simulink model "main_RI_LIEKF_GNSSOutrage"  (R2023a)
settings: Solver=FixedStepAuto  StartTime=0.0  StopTime=220  FixedStep=0.01  RelTol=1e-3
InitFcn:
  | initNavigation0612_AOA;
values from neighbouring files (symbols this model uses):
  CF_enable = 0    [initNavigation.m]
  dt = 0.01    [initNavigation.m]
  dtDelay = -0.03    [initNavigation.m]
  g0 = 9.795    [initNavigation.m]
  gam0_rad = 0/57.3    (= 0)    [initNavigation.m]
  GNSSoutragetime = 90    [initNavigation.m]
  H_sensor_type = 0    [initNavigation.m]
  KF_enable = 1    [initNavigation.m]
  P0 = diag([1*ones(3,1);0.01*ones(3,1);0.1*ones(3,1);0.001*ones(3,1);0.00001*ones(3,1)])    [initNavigation.m]
  P0_RIEKF = diag([1*ones(3,1);0.01*ones(3,1);0.1*ones(3,1);0.001*ones(3,1);0.00001*ones(3,1);      0.01*ones(3,1);[0;2;2]/57.3;[0.1;0.1;0.1]])^2    [initNavigation.m]
  pd0 = 0    [initNavigation.m]
  pe0 = 0    [initNavigation.m]
  phi0_rad = 0/57.3    (= 0)    [initNavigation.m]
  pn0 = 0    [initNavigation.m]
  psi = -178    [initNavigation.m]
  psi0_rad = 0/57.3    (= 0)    [initNavigation.m]
  state_dim = 24    [initNavigation.m]
  Time = 0:0.01:(size(traindata.AttackAngle,1) - 1)*0.01    [NNLiftCoefficientFit.m]
  vd0 = 0    [initNavigation.m]
  ve0 = 0    [initNavigation.m]
  vn0 = 0    [initNavigation.m]
undefined symbols (not defined in the file or in its folder): DiscIntNeverNeededParam, Discrete, INS_CONST, INS_EXPORT, INS_PARAM, magnitude, p, param, pInitialization, sys
libraries: simulink_extras x94, simulink x82, dspstat3 x70, sharedtransform x60, ctrlSharedLib x36, sharedTrackingLibrary x22, matrix_library x15, FMT_Model_Lib x13, deeplib x8, dspsolvers x4, vrlib x4, aerolibconvert2 x1
(part 20 of 28)

== system main_RI_LIEKF_GNSSOutrage/State estimation/distribute CF/AHRS/Init_Q0/Horizontal_attitude ==
  note: gamma
  note: fai
  accl_mean_B_m/s_LPF : Inport  PortDimensions=3
  Magn_mean_B_guess_LPF : Inport  Port=2
  Enable : EnablePort
  Add : Sum  Inputs=+-
  Add1 : Sum
  Add2 : Sum
  Add3 : Sum
  Asin : Trigonometry  Operator=asin
  Atan2 : Trigonometry  Operator=atan2
  Data Type Conversion : DataTypeConversion  SaturateOnIntegerOverflow=off  RndMeth=Floor
  Deal with zero : Subsystem
  Degrees to Radians : simulink_extras/Transformations/Degrees to Radians
  Degrees to Radians1 : simulink_extras/Transformations/Degrees to Radians
  Demux : Demux  Outputs=3
  Divide : Product  Inputs=*/  OutDataTypeStr=single
  Gain1 : Gain  Gain=-1
  Gain2 : Gain  Gain=-1
  Magnetic declination : Constant  Value=param.fusion.magDeclDeg  OutDataTypeStr=single
  Magnetic declination1 : Constant  Value=param.control.MagnheadingCorrection  OutDataTypeStr=uint8
  Math Function : Math  Operator=magnitude^2  SignedPower=on
  Mux : Mux  Inputs=3
  Mux1 : Mux  Inputs=3
  Mux3 : Mux  Inputs=3
  Product : Product  Multiplication=Matrix(*)
  Quaternions to Direction Cosine Matrix : sharedtransform/Quaternions to  Direction Cosine Matrix  aMode=aMode
  Rotation Angles to Quaternions : sharedtransform/Rotation Angles to Quaternions  rotationOrder=ZYX  aMode=aMode
  Rotation Angles to Quaternions1 : sharedtransform/Rotation Angles to Quaternions  rotationOrder=ZYX  aMode=aMode
  Scope : Scope
  Scope1 : Scope
  Selector : Selector  InputPortWidth=3  IndexOptions=Index vector (dialog)  Indices=[2]  OutputSizes=1
  Selector1 : Selector  InputPortWidth=3  IndexOptions=Index vector (dialog)  Indices=[1]  OutputSizes=1
  Sqrt : Sqrt
  Sum of Elements : Sum  Inputs=+
  Switch : Switch  Threshold=0.5  SaturateOnIntegerOverflow=off  InputSameDT=off
  Terminator : Terminator
  Transpose : Math  Operator=transpose  SignedPower=on
  Trigonometric Function1 : Trigonometry  Operator=atan2
  psi_zero : Constant  Value=psi  OutDataTypeStr=single
  psi_zero1 : Constant  Value=psi0_rad  OutDataTypeStr=single
  psi_zero2 : Constant  Value=phi0_rad  OutDataTypeStr=single
  psi_zero3 : Constant  Value=gam0_rad  OutDataTypeStr=single
  quat_0 : Outport  PortDimensions=4
  wires:
  Data Type Conversion/1 -> Scope/1
  Rotation Angles to Quaternions1/1 -> Switch/1
  Switch/1 -> quat_0/1, Scope1/1
  Magnetic declination1/1 -> Switch/2, Data Type Conversion/1
  Degrees to Radians/1 -> Terminator/1
  Add1/1 -> Mux1/1
  Gain1/1 -> Mux/3, Trigonometric Function1/2
  Transpose/1 -> Product/1
  Mux3/1 -> Rotation Angles to Quaternions1/1
  Add/1 -> Mux3/1  "psi_calbymag"
  Magnetic declination/1 -> Degrees to Radians/1
  Atan2/1 -> Add/2
  Selector/1 -> Atan2/1  "magE"
  Selector1/1 -> Atan2/2  "magN"
  Product/1 -> Selector1/1, Selector/1  "magNED"
  Magn_mean_B_guess_LPF/1 -> Product/2
  Quaternions to Direction Cosine Matrix/1 -> Transpose/1
  Rotation Angles to Quaternions/1 -> Quaternions to Direction Cosine Matrix/1, Switch/3  "q0_no_yaw"
  Add3/1 -> Mux3/3, Mux1/3
  Add2/1 -> Mux1/2, Mux3/2
  psi_zero/1 -> Degrees to Radians1/1
  Mux1/1 -> Rotation Angles to Quaternions/1
  Math Function/1 -> Sum of Elements/1
  Mux/1 -> Math Function/1
  Divide/1 -> Asin/1
  Sum of Elements/1 -> Sqrt/1
  Demux/3 -> Gain1/1
  Demux/2 -> Trigonometric Function1/1, Mux/1
  Demux/1 -> Mux/2, Divide/1
  Trigonometric Function1/1 -> Gain2/1
  Deal with zero/1(Out1) -> Divide/2
  Sqrt/1 -> Deal with zero/1(In1)
  accl_mean_B_m/s_LPF/1 -> Demux/1
  psi_zero1/1 -> ?
  Degrees to Radians1/1 -> Add1/2
  psi_zero2/1 -> ?
  Asin/1 -> Add2/2
  psi_zero3/1 -> ?
  Gain2/1 -> Add3/2

== system main_RI_LIEKF_GNSSOutrage/State estimation/distribute CF/AHRS/Init_Q0/Subsystem ==
  data : Inport
  Buffer : Buffer  N=50  V=49  OutputFrames=off
  Buffer1 : Buffer  N=50  V=49  OutputFrames=off
  Buffer2 : Buffer  N=50  V=49  ic=-g0  OutputFrames=off
  Demux : Demux  Outputs=3
  Mean4 : dspstat3/Mean  run=off  reset_popup=None  directionMode=Entire input  dimension=3  roiEnable=off  roiType=Rectangles  roiPortion=Entire ROI  roiOutput=Individual statistics for each ROI  roiFlag=off  roundingMode=Floor  overflowMode=off  outputDataTypeStr=Inherit: Same as accumulator  outputMin=[]  outputMax=[]  outputLastDataTypeStr=Inherit: Same as accumulator
  Mean5 : dspstat3/Mean  run=off  reset_popup=None  directionMode=Entire input  dimension=3  roiEnable=off  roiType=Rectangles  roiPortion=Entire ROI  roiOutput=Individual statistics for each ROI  roiFlag=off  roundingMode=Floor  overflowMode=off  outputDataTypeStr=Inherit: Same as accumulator  outputMin=[]  outputMax=[]  outputLastDataTypeStr=Inherit: Same as accumulator
  Mean6 : dspstat3/Mean  run=off  reset_popup=None  directionMode=Entire input  dimension=3  roiEnable=off  roiType=Rectangles  roiPortion=Entire ROI  roiOutput=Individual statistics for each ROI  roiFlag=off  roundingMode=Floor  overflowMode=off  outputDataTypeStr=Inherit: Same as accumulator  outputMin=[]  outputMax=[]  outputLastDataTypeStr=Inherit: Same as accumulator
  Scope : Scope  NumInputPorts=2
  Vector Concatenate : Concatenate  NumInputs=3
  mean_data : Outport
  wires:
  data/1 -> Demux/1, Scope/1
  Vector Concatenate/1 -> mean_data/1, Scope/2
  Mean4/1 -> Vector Concatenate/1
  Demux/3 -> Buffer2/1
  Buffer1/1 -> Mean5/1  "fby_buff"
  Demux/1 -> Buffer/1
  Buffer2/1 -> Mean6/1  "fbz_buff"
  Mean5/1 -> Vector Concatenate/2
  Buffer/1 -> Mean4/1  "fbx_buff"
  Demux/2 -> Buffer1/1
  Mean6/1 -> Vector Concatenate/3

== system main_RI_LIEKF_GNSSOutrage/State estimation/distribute CF/AHRS/Init_Q0/Subsystem1 ==
  data : Inport
  Buffer : Buffer  N=50  V=49  OutputFrames=off
  Buffer1 : Buffer  N=50  V=49  OutputFrames=off
  Buffer2 : Buffer  N=50  V=49  OutputFrames=off
  Demux : Demux  Outputs=3
  Mean4 : dspstat3/Mean  run=off  reset_popup=None  directionMode=Entire input  dimension=3  roiEnable=off  roiType=Rectangles  roiPortion=Entire ROI  roiOutput=Individual statistics for each ROI  roiFlag=off  roundingMode=Floor  overflowMode=off  outputDataTypeStr=Inherit: Same as accumulator  outputMin=[]  outputMax=[]  outputLastDataTypeStr=Inherit: Same as accumulator
  Mean5 : dspstat3/Mean  run=off  reset_popup=None  directionMode=Entire input  dimension=3  roiEnable=off  roiType=Rectangles  roiPortion=Entire ROI  roiOutput=Individual statistics for each ROI  roiFlag=off  roundingMode=Floor  overflowMode=off  outputDataTypeStr=Inherit: Same as accumulator  outputMin=[]  outputMax=[]  outputLastDataTypeStr=Inherit: Same as accumulator
  Mean6 : dspstat3/Mean  run=off  reset_popup=None  directionMode=Entire input  dimension=3  roiEnable=off  roiType=Rectangles  roiPortion=Entire ROI  roiOutput=Individual statistics for each ROI  roiFlag=off  roundingMode=Floor  overflowMode=off  outputDataTypeStr=Inherit: Same as accumulator  outputMin=[]  outputMax=[]  outputLastDataTypeStr=Inherit: Same as accumulator
  Vector Concatenate : Concatenate  NumInputs=3
  mean_data : Outport
  wires:
  Mean6/1 -> Vector Concatenate/3
  Demux/2 -> Buffer1/1
  Buffer/1 -> Mean4/1  "fbx_buff"
  Mean5/1 -> Vector Concatenate/2
  Buffer2/1 -> Mean6/1  "fbz_buff"
  Demux/1 -> Buffer/1
  Buffer1/1 -> Mean5/1  "fby_buff"
  Demux/3 -> Buffer2/1
  Mean4/1 -> Vector Concatenate/1
  Vector Concatenate/1 -> mean_data/1
  data/1 -> Demux/1

== system main_RI_LIEKF_GNSSOutrage/State estimation/distribute CF/AHRS/att_update/uniformization ==
  Q i : Inport  PortDimensions=4
  Constant : Constant  Value=1e-20
  Dot Product1 : DotProduct  OutDataTypeStr=Inherit: Inherit via internal rule
  Math Function : Math  Operator=sqrt  SignedPower=on
  Product : Product  Inputs=*/  SaturateOnIntegerOverflow=on  OutDataTypeStr=Inherit: Same as first input
  Sum : Sum  Inputs=|++  SaturateOnIntegerOverflow=on
  Q o : Outport
  wires:
  Sum/1 -> Product/2
  Constant/1 -> Sum/2
  Product/1 -> Q o/1
  Math Function/1 -> Sum/1
  Dot Product1/1 -> Math Function/1
  Q i/1 -> Product/1, Dot Product1/1, Dot Product1/2

== system main_RI_LIEKF_GNSSOutrage/State estimation/distribute CF/Translation_estimate/Rxy_Horizontal_estimation/Integrator_R_Horizontal ==
  Vn : Inport
  dR : Inport  Port=2
  Sensor_data2 : Inport  Port=3
  Bus Selector : BusSelector  OutputSignals=QGC_sensor_reinit,GPS_Data.pos_N_gps,GPS_Data.pos_E_gps
  Delay : Delay  DelayLength=1  InitialConditionSource=Input port  ExternalReset=Rising
      settings: InputPortMap=u0,r5,p4
  Gain : Gain  Gain=0.8
  Gain2 : Gain  Gain=dt  SaturateOnIntegerOverflow=on  OutDataTypeStr=Inherit: Same as input  ParamDataTypeStr=Inherit: Same as input
  Mux : Mux  Inputs=2
  Sum : Sum  Inputs=|++-
  R_n&e : Outport
  wires:
  Gain/1 -> Sum/3
  dR/1 -> Gain/1
  Vn/1 -> Gain2/1
  Gain2/1 -> Sum/1
  Sum/1 -> R_n&e/1, Delay/1
  Sensor_data2/1 -> Bus Selector/1
  Bus Selector/1 -> Delay/2  "<QGC_sensor_reinit>"
  Bus Selector/2 -> Mux/1  "<pos_N_gps>"
  Bus Selector/3 -> Mux/2  "<pos_E_gps>"
  Mux/1 -> Delay/3
  Delay/1 -> Sum/2

== system main_RI_LIEKF_GNSSOutrage/State estimation/distribute CF/Translation_estimate/Rxy_Horizontal_estimation/Rxy_kalman filter2 ==
  X : Inport
  Z : Inport  Port=2
  Enable : Inport  Port=3
  Constant : Constant  Value=F  OutDataTypeStr=single
  Constant1 : Constant  Value=Q  OutDataTypeStr=single
  Constant2 : Constant  Value=R  OutDataTypeStr=single
  Constant3 : Constant  Value=P0  OutDataTypeStr=single
  Constant4 : Constant  Value=H  OutDataTypeStr=single
  Vxy kalman filter : Subsystem  TreatAsAtomicUnit=on
  XOut : Outport
  wires:
  Enable/1 -> Vxy kalman filter/9(Enable)
  Vxy kalman filter/1(XOut) -> XOut/1
  Constant1/1 -> Vxy kalman filter/5(Q)
  Constant4/1 -> Vxy kalman filter/4(H)
  Constant2/1 -> Vxy kalman filter/6(R)
  Constant3/1 -> Vxy kalman filter/8(P0)
  Z/1 -> Vxy kalman filter/1(Z)
  Constant/1 -> Vxy kalman filter/3(G), Vxy kalman filter/2(F)
  X/1 -> Vxy kalman filter/7(X)

== system main_RI_LIEKF_GNSSOutrage/State estimation/distribute CF/Translation_estimate/V_Horizontal_estimation/Integrator_V_Horizontal ==
  An : Inport
  dv : Inport  Port=2
  Sensor_data2 : Inport  Port=3
  Bus Selector : BusSelector  OutputSignals=QGC_sensor_reinit,GPS_Data.vn_gps,GPS_Data.ve_gps
  Delay : Delay  DelayLength=1  InitialConditionSource=Input port  ExternalReset=Rising
      settings: InputPortMap=u0,r5,p4
  Gain : Gain
  Gain2 : Gain  Gain=dt  SaturateOnIntegerOverflow=on  OutDataTypeStr=Inherit: Same as input  ParamDataTypeStr=Inherit: Same as input
  Mux : Mux  Inputs=2
  Scope : Scope
  Sum : Sum  Inputs=|++-
  V_n&e : Outport
  wires:
  Gain/1 -> Sum/3, Scope/1
  dv/1 -> Gain/1
  Delay/1 -> Sum/2
  Mux/1 -> Delay/3
  Bus Selector/3 -> Mux/2  "<ve_gps>"
  Bus Selector/2 -> Mux/1  "<vn_gps>"
  Bus Selector/1 -> Delay/2  "<QGC_sensor_reinit>"
  Sensor_data2/1 -> Bus Selector/1
  Sum/1 -> Delay/1, V_n&e/1
  Gain2/1 -> Sum/1
  An/1 -> Gain2/1

== system main_RI_LIEKF_GNSSOutrage/State estimation/distribute CF/Translation_estimate/V_Horizontal_estimation/Rxy_kalman filter1 ==
  X : Inport
  Z : Inport  Port=2
  Enable : Inport  Port=3
  Constant : Constant  Value=F  OutDataTypeStr=single
  Constant1 : Constant  Value=Q  OutDataTypeStr=single
  Constant2 : Constant  Value=R  OutDataTypeStr=single
  Constant3 : Constant  Value=P0  OutDataTypeStr=single
  Constant4 : Constant  Value=H  OutDataTypeStr=single
  Vxy kalman filter : Subsystem  TreatAsAtomicUnit=on
  XOut : Outport
  wires:
  X/1 -> Vxy kalman filter/7(X)
  Constant/1 -> Vxy kalman filter/2(F), Vxy kalman filter/3(G)
  Z/1 -> Vxy kalman filter/1(Z)
  Constant3/1 -> Vxy kalman filter/8(P0)
  Constant2/1 -> Vxy kalman filter/6(R)
  Constant4/1 -> Vxy kalman filter/4(H)
  Constant1/1 -> Vxy kalman filter/5(Q)
  Vxy kalman filter/1(XOut) -> XOut/1
  Enable/1 -> Vxy kalman filter/9(Enable)

== system main_RI_LIEKF_GNSSOutrage/State estimation/distribute CF/distribute CF/AHRS1/Bus_Constructor ==
  RF_Data : Inport
  att_quat : Inport  Port=2
  DCM_OB : Inport  Port=3
  bias_g : Inport  Port=4
  Sensor_Data : Inport  Port=5
  Bus Creator : BusCreator  Inputs=12
  Bus Selector : BusSelector  OutputSignals=IMU_Data.gyr_B_radPs,IMU_Data.acc_B_mPs2
  Bus Selector1 : BusSelector  OutputSignals=att_reset
  Bus Selector2 : BusSelector  OutputSignals=standstill
  Euler_Angle : Subsystem
  Math Function : Math  Operator=transpose  SignedPower=on
  Psi To DCM : FMT_Model_Lib/Transformation/Psi To DCM
  Signal Conversion{,1..4} (5 alike) : SignalConversion  OverrideOpt=off
  Rotation_Data : Outport
  wires:
  Bus Selector1/1 -> Signal Conversion4/1  "<att_reset>"
  Signal Conversion/1 -> Bus Creator/11  "acc_B_mPs2"
  Euler_Angle/1(phi_rad) -> Bus Creator/2  "phi_rad"
  Euler_Angle/2(theta_rad) -> Bus Creator/3  "theta_rad"
  Euler_Angle/3(psi_rad) -> Psi To DCM/1, Bus Creator/4  "psi_rad"
  Sensor_Data/1 -> Bus Selector/1
  Bus Selector2/1 -> Signal Conversion1/1  "<standstill>"
  Bus Creator/1 -> Rotation_Data/1
  bias_g/1 -> Signal Conversion3/1
  Math Function/1 -> Bus Creator/7  "M_BO"
  DCM_OB/1 -> Math Function/1, Bus Creator/8  "M_OB"
  att_quat/1 -> Euler_Angle/1(att_quat), Bus Creator/6  "att_quat"
  Psi To DCM/1 -> Bus Creator/5  "M_CO"
  Signal Conversion1/1 -> Bus Creator/12  "standstill"
  Bus Selector/2 -> Signal Conversion/1  "<acc_B_mPs2>"
  Signal Conversion2/1 -> Bus Creator/10  "gyr_B_radPs"
  Signal Conversion3/1 -> Bus Creator/9  "bias_g"
  RF_Data/1 -> Bus Selector2/1, Bus Selector1/1  "att_reset"
  Bus Selector/1 -> Signal Conversion2/1  "<gyr_B_radPs>"
  Signal Conversion4/1 -> Bus Creator/1  "att_reset"

== system main_RI_LIEKF_GNSSOutrage/State estimation/distribute CF/distribute CF/AHRS1/Correct ==
  Rotation_Data : Inport
  Sensor_Data : Inport  Port=2
  RF_Data : Inport  Port=3
  Attitude_Correction : Subsystem
  Bus Selector : BusSelector  OutputSignals=standstill
  Bus Selector1 : BusSelector  OutputSignals=IMU_Data
  Gyro_Bias_Correction : Subsystem
  att_B_correction : Outport
  bias_g_B_correction : Outport  Port=2
  wires:
  Gyro_Bias_Correction/1(bias_g_B_correction) -> bias_g_B_correction/1
  Bus Selector1/1 -> Gyro_Bias_Correction/2(IMU_Data)  "<IMU_Data>"
  RF_Data/1 -> Bus Selector/1
  Attitude_Correction/1(att_B_correction) -> att_B_correction/1, Gyro_Bias_Correction/1(att_B_correction)
  Sensor_Data/1 -> Attitude_Correction/1(Sensor_Data), Bus Selector1/1
  Rotation_Data/1 -> Attitude_Correction/2(Rotation_Data)
  Bus Selector/1 -> Attitude_Correction/3(standstill)  "<standstill>"

== system main_RI_LIEKF_GNSSOutrage/State estimation/distribute CF/distribute CF/AHRS1/Update ==
  att_B_correction : Inport
  bias_g_correction : Inport  Port=2
  RF_Data : Inport  Port=3
  Sensor_Data : Inport  Port=4
  Attitude_Update : Subsystem
  Bus Selector : BusSelector  OutputSignals=IMU_Data.gyr_B_radPs
  Bus Selector1 : BusSelector  OutputSignals=att_reset,quat_0
  Gyro_Bias_Update : Subsystem
  Sum2 : Sum  Inputs=|++
  att_quat : Outport
  DCM_OB : Outport  Port=2
  bias_g : Outport  Port=3
  wires:
  Sensor_Data/1 -> Bus Selector/1
  Gyro_Bias_Update/1(gyr_B_correction) -> Sum2/2
  att_B_correction/1 -> Sum2/1
  Sum2/1 -> Attitude_Update/3(att_B_correction)
  Bus Selector/1 -> Gyro_Bias_Update/2(gyr_B_radPs)  "<gyr_B_radPs>"
  bias_g_correction/1 -> Gyro_Bias_Update/1(bias_g_correction)
  Attitude_Update/1(att_quat) -> att_quat/1
  Attitude_Update/2(DCM_OB) -> DCM_OB/1
  Gyro_Bias_Update/2(bias_g) -> bias_g/1
  RF_Data/1 -> Bus Selector1/1  "att_reset"
  Bus Selector1/1 -> Attitude_Update/1(att_reset)  "<att_reset>"
  Bus Selector1/2 -> Attitude_Update/2(quat_0)  "<quat_0>"

== system main_RI_LIEKF_GNSSOutrage/State estimation/distribute CF/distribute CF/Bus_Constructor/Euler_Angle ==
  att_quat : Inport
  Demux : Demux  Outputs=3
  Quaternions to Rotation Angles : sharedtransform/Quaternions to Rotation Angles  rotationOrder=ZYX  aMode=aMode
  phi_rad : Outport
  theta_rad : Outport  Port=2
  psi_rad : Outport  Port=3
  wires:
  Demux/1 -> phi_rad/1
  Demux/2 -> theta_rad/1
  Demux/3 -> psi_rad/1
  att_quat/1 -> Quaternions to Rotation Angles/1
  Quaternions to Rotation Angles/1 -> Demux/1

== system main_RI_LIEKF_GNSSOutrage/State estimation/distribute CF/distribute CF/Bus_Constructor/Subsystem1 ==
  psi : Inport
  Gain : Gain  Gain=-1
  Subsystem : Subsystem
  DCMz : Outport
  wires:
  psi/1 -> Gain/1
  Gain/1 -> Subsystem/1(psi)
  Subsystem/1(DCMz) -> DCMz/1

== system main_RI_LIEKF_GNSSOutrage/State estimation/distribute CF/distribute CF/Correct/Attitude_Correction ==
  note: N系到B系
  Sensor_Data : Inport
  Rotation_Data : Inport  Port=2
  Attitude_Correct : Subsystem
  Bus Selector2 : BusSelector  OutputSignals=M_BO
  Mag_Correct : Subsystem
  Multiply : Product  Multiplication=Matrix(*)
  Scope : Scope
  Sum : Sum  Inputs=|++
  att_B_correction : Outport
  wires:
  Multiply/1 -> att_B_correction/1
  Rotation_Data/1 -> Bus Selector2/1, Attitude_Correct/2(Rotation_Data), Mag_Correct/1(Rotation_Data)
  Sensor_Data/1 -> Mag_Correct/2(Sensor_Data), Attitude_Correct/1(Sensor_Data)
  Bus Selector2/1 -> Multiply/1  "<M_BO>"
  Sum/1 -> Multiply/2
  Attitude_Correct/1(att_corr_O) -> Sum/1
  Mag_Correct/1(mag_corr_O) -> Scope/1  "mag_corr_O"

== system main_RI_LIEKF_GNSSOutrage/State estimation/distribute CF/distribute CF/Correct/Subsystem2 ==
  note: 零速判断
  note: 误差角r
  note: 误差角速度r‘
  Sensor_Data : Inport
  att_B_correction : Inport  Port=2
  Abs : Abs  SaturateOnIntegerOverflow=off
  Bus Selector1 : BusSelector  OutputSignals=IMU_Data.accl_B_m/s2_LPF
  Compare To Constant : simulink/Logic and Bit Operations/Compare To Constant  relop=<=  const=1  OutDataTypeStr=boolean
  Constant : Constant  Value=g0  OutDataTypeStr=single
  Data Type Conversion : DataTypeConversion  OutDataTypeStr=single  SaturateOnIntegerOverflow=off  RndMeth=Floor
  Gain1 : Gain  Gain=gbias_correct_gain
  MX Product1 : Product  RndMeth=Simplest
  Saturation2 : Saturate  UpperLimit=0.1/180*pi  LowerLimit=-0.1/180*pi
  Scope : Scope
  Scope1 : Scope  NumInputPorts=2
  Subtract : Sum  Inputs=+-
  norm : Subsystem
  低通滤波 : Subsystem  mask{fc=5, zeta=0.707}
      mask prompts: fc "Cut-off frequence"; zeta "Damping factor"
      mask DialogControl ParameterGroupVar Prompt: 参数
  bias_g_B_correction : Outport
  wires:
  Sensor_Data/1 -> Bus Selector1/1
  Saturation2/1 -> bias_g_B_correction/1  "bias_g_correction"
  Constant/1 -> Subtract/2
  Compare To Constant/1 -> Data Type Conversion/1
  att_B_correction/1 -> MX Product1/1
  Data Type Conversion/1 -> Scope/1, MX Product1/2
  MX Product1/1 -> Scope1/1, 低通滤波/1(u)
  Subtract/1 -> Abs/1
  norm/1(Out1) -> Subtract/1
  Bus Selector1/1 -> norm/1(In1)  "<accl_B_m/s2_LPF>"
  Abs/1 -> Compare To Constant/1
  Gain1/1 -> Saturation2/1
  低通滤波/1(y) -> Scope1/2, Gain1/1

== system main_RI_LIEKF_GNSSOutrage/State estimation/distribute CF/distribute CF/Translation_estimate/Rxy_Horizontal_estimation ==
  Vn : Inport
  Enable : Inport  Port=2
  Sensor_data2 : Inport  Port=3
  Cbn : Inport  Port=4
  Add1 : Sum  Inputs=+-
  Bus Selector1 : BusSelector  OutputSignals=GPS_Data.pos_N_gps,GPS_Data.pos_E_gps
  Data Store Memory : DataStoreMemory  DataStoreName=GPS_enable_CF  WriteAfterWriteMsg=warning  ShowAdditionalParam=off
  Data Store Read : DataStoreRead  DataStoreName=GPS_enable_CF  IndexOptions=Index vector (dialog)  Indices=1  OutputSizes=1
  Data Store Write : DataStoreWrite  DataStoreName=GPS_enable_CF  IndexOptions=Index vector (dialog)  Indices=1  OutputSizes=1
  Delay1 : Delay  DelayLength=1
  Integrator_R_Horizontal : Subsystem
  Mux1 : Mux  Inputs=2
  Rxy_kalman filter2 : Subsystem  mask{F=diag([-0.1,-0.1,-0.01,-0.01]), H=[1,0,-1,0;0,1,0,-1], Q=diag([1,1,0.1,0.1]), R=diag([0.05,0.05]), P0=diag([0.8,0.8,0.2,0.2])}
      mask prompts: F "状态转移矩阵：F"; H "观测转移矩阵：H"; Q "预测噪声协方差矩阵：Q"; R "量测噪声协方差矩阵：R"; P0 "初始协方差矩阵：P0"
      mask DialogControl DescTextVar Prompt: Kalman Filter
  Scope : Scope
  Scope1 : Scope  NumInputPorts=2
  Scope5 : Scope
  Selector1 : Selector  InputPortWidth=4  IndexOptions=Index vector (dialog)  Indices=[1 2]  OutputSizes=1
  Subsystem : Subsystem
  R_n&e : Outport
  wires:
  Vn/1 -> Integrator_R_Horizontal/1(Vn)
  Add1/1 -> Rxy_kalman filter2/2(Z)
  Rxy_kalman filter2/1(XOut) -> Scope/1, Delay1/1
  Bus Selector1/1 -> Mux1/1  "<pos_N_gps>"
  Integrator_R_Horizontal/1(R_n&e) -> R_n&e/1
  Bus Selector1/2 -> Mux1/2  "<pos_E_gps>"
  Sensor_data2/1 -> Bus Selector1/1, Integrator_R_Horizontal/3(Sensor_data2)
  Delay1/1 -> Rxy_kalman filter2/1(X), Selector1/1
  Mux1/1 -> Scope1/2, Add1/2
  Selector1/1 -> Integrator_R_Horizontal/2(dR)
  Cbn/1 -> Integrator_R_Horizontal/4(Cbn)
  Integrator_R_Horizontal/2(R_n&eL) -> Scope1/1, Add1/1
  Subsystem/1(flag) -> Scope5/1, Data Store Write/1
  Data Store Read/1 -> Rxy_kalman filter2/3(Enable)

== system main_RI_LIEKF_GNSSOutrage/State estimation/distribute CF/distribute CF/Translation_estimate/V_Horizontal_estimation ==
  note: 0530改：
      | 加入GPStype限制
  An : Inport
  Sensor_data2 : Inport  Port=2
  Add : Sum  Inputs=+-
  Bus Selector2 : BusSelector  OutputSignals=GPS_Data.vn_gps,GPS_Data.ve_gps,GPS_Data.fixtype_gps
  Compare To Constant : simulink/Logic and Bit Operations/Compare To Constant  relop=>=  const=1  OutDataTypeStr=boolean
  Delay : Delay  DelayLength=1
  Detect Change : simulink/Logic and Bit Operations/Detect Change  vinit=0  OutDataTypeStr=boolean
  Integrator_V_Horizontal : Subsystem
  Logical Operator : Logic  AllPortsSameDT=off  OutDataTypeStr=boolean
  Mux : Mux  Inputs=2
  Rxy_kalman filter1 : Subsystem  mask{F=diag([-0.1,-0.1,-0.01,-0.01]), H=[1,0,-1,0;0,1,0,-1], Q=diag([1,1,0.1,0.1]), R=diag([0.1,0.1]), P0=diag([0.8,0.8,0.5,0.5])}
      mask prompts: F "状态转移矩阵：F"; H "观测转移矩阵：H"; Q "预测噪声协方差矩阵：Q"; R "量测噪声协方差矩阵：R"; P0 "初始协方差矩阵：P0"
      mask DialogControl DescTextVar Prompt: Kalman Filter
  Scope : Scope  NumInputPorts=2
  Scope1 : Scope
  Selector : Selector  InputPortWidth=4  IndexOptions=Index vector (dialog)  Indices=[1 2]  OutputSizes=1
  vxy_estimout : Outport
  V_n&e : Outport  Port=2
  GPS_v_enable : Outport  Port=3
  wires:
  Logical Operator/1 -> Rxy_kalman filter1/3(Enable), GPS_v_enable/1, Scope1/1
  Compare To Constant/1 -> Logical Operator/2
  Detect Change/1 -> Logical Operator/1
  Bus Selector2/3 -> Compare To Constant/1  "<fixtype_gps>"
  Sensor_data2/1 -> Integrator_V_Horizontal/3(Sensor_data2), Bus Selector2/1
  An/1 -> Integrator_V_Horizontal/1(An)
  Add/1 -> Rxy_kalman filter1/2(Z)
  Integrator_V_Horizontal/1(V_n&e) -> Add/1, Scope/1, vxy_estimout/1, V_n&e/1
  Rxy_kalman filter1/1(XOut) -> Delay/1
  Bus Selector2/2 -> Mux/2  "<ve_gps>"
  Mux/1 -> Add/2, Scope/2
  Bus Selector2/1 -> Detect Change/1, Mux/1  "<vn_gps>"
  Selector/1 -> Integrator_V_Horizontal/2(dv)
  Delay/1 -> Rxy_kalman filter1/1(X), Selector/1

== system main_RI_LIEKF_GNSSOutrage/State estimation/distribute CF/distribute CF/Translation_estimate/translate to N ==
  RotationData : Inport
  Sensor_data : Inport  Port=2
  Bus Selector2 : BusSelector  OutputSignals=IMU_Data.accl_B_m/s2_LPF
  Bus Selector3 : BusSelector  OutputSignals=M_OB
  Product : Product  Multiplication=Matrix(*)
  Selector : Selector  InputPortWidth=3  IndexOptions=Index vector (dialog)  Indices=[1 2]  OutputSizes=1
  Selector1 : Selector  InputPortWidth=3  IndexOptions=Index vector (dialog)  Indices=[3]  OutputSizes=1
  accel_Horizontal_predict : Outport
  accel_Vertical_predict : Outport  Port=2
  wires:
  Selector1/1 -> accel_Vertical_predict/1
  Selector/1 -> accel_Horizontal_predict/1
  Product/1 -> Selector/1, Selector1/1
  Sensor_data/1 -> Bus Selector2/1
  Bus Selector3/1 -> Product/1  "<M_OB>"
  Bus Selector2/1 -> Product/2  "<accl_B_m/s2_LPF>"
  RotationData/1 -> Bus Selector3/1

== system main_RI_LIEKF_GNSSOutrage/State estimation/distribute CF/distribute CF/Update/Attitude_Update ==
  att_reset : Inport
  quat_0 : Inport  Port=2
  att_B_correction : Inport  Port=3
  Delay : Delay  DelayLength=1  InitialConditionSource=Input port  ExternalReset=Rising
      settings: InputPortMap=u0,r5,p4
  Gain : Gain  Gain=dt
  QuatMult1 : MATLAB Function  TreatAsAtomicUnit=on
  Quaternions to Direction Cosine Matrix1 : sharedtransform/Quaternions to  Direction Cosine Matrix  aMode=aMode
  Transpose1 : Math  Operator=transpose  SignedPower=on
  rv2q : MATLAB Function  TreatAsAtomicUnit=on
  uniformization1 : Subsystem
  att_quat : Outport
  DCM_OB : Outport  Port=2
  wires:
  Transpose1/1 -> DCM_OB/1  "DCM_b_n"
  rv2q/1(quaternion) -> QuatMult1/2(quatB)
  uniformization1/1(Q o) -> att_quat/1, Delay/1, Quaternions to Direction Cosine Matrix1/1  "q_update"
  Gain/1 -> rv2q/1(rotVec)  "correctedDelAng"
  Delay/1 -> QuatMult1/1(quatA)
  att_B_correction/1 -> Gain/1
  Quaternions to Direction Cosine Matrix1/1 -> Transpose1/1
  QuatMult1/1(quatOut) -> uniformization1/1(Q i)  "q_update"
  att_reset/1 -> Delay/2
  quat_0/1 -> Delay/3

== system main_RI_LIEKF_GNSSOutrage/State estimation/distribute CF/distribute CF/Update/Gyro_Bias_Update ==
  bias_g_correction : Inport
  gyr_B_radPs : Inport  Port=2
  Discrete-Time Integrator2 : DiscreteIntegrator  gainval=1  SampleTime=-1  LimitOutput=on  UpperSaturationLimit=45/180*pi  LowerSaturationLimit=-45/180*pi  ICPrevOutput=DiscIntNeverNeededParam  ICPrevScaledInput=DiscIntNeverNeededParam
  Sum1 : Sum  Inputs=++|
  gyr_B_correction : Outport
  bias_g : Outport  Port=2
  wires:
  Discrete-Time Integrator2/1 -> Sum1/1, bias_g/1
  gyr_B_radPs/1 -> Sum1/2
  Sum1/1 -> gyr_B_correction/1
  bias_g_correction/1 -> Discrete-Time Integrator2/1

== system main_RI_LIEKF_GNSSOutrage/State estimation/distribute CF/distribute CF/初始化/Attitude_Reset ==
  Sensor_Data : Inport
  Bus Selector : BusSelector  OutputSignals=IMU_Data.accl_B_m/s2_LPF
  Bus Selector1 : BusSelector  OutputSignals=GPS_Data.fixtype_gps
  Detect Rise Positive : simulink/Logic and Bit Operations/Detect Rise Positive  vinit=0  OutDataTypeStr=boolean
  Interval Test : simulink/Logic and Bit Operations/Interval Test  IntervalClosedRight=on  uplimit=g0+0.5  IntervalClosedLeft=on  lowlimit=g0-0.5  OutDataTypeStr=boolean
  Logical Operator : Logic  AllPortsSameDT=off  OutDataTypeStr=boolean
  Logical Operator2 : Logic  Operator=OR  AllPortsSameDT=off  OutDataTypeStr=boolean
  Reset Heading : Subsystem
  norm : Subsystem
  sample_valid : Subsystem
  att_reset : Outport
  wires:
  sample_valid/1(sample_valid) -> Logical Operator/1, Detect Rise Positive/1
  norm/1(Out1) -> Interval Test/1
  Interval Test/1 -> sample_valid/1(valid)
  Sensor_Data/1 -> Bus Selector1/1, Bus Selector/1
  Bus Selector/1 -> norm/1(In1)  "<accl_B_m/s2_LPF>"
  Detect Rise Positive/1 -> Logical Operator2/1
  Logical Operator/1 -> Logical Operator2/2
  Logical Operator2/1 -> att_reset/1
  Bus Selector1/1 -> Reset Heading/1(GPS_valid)  "<fixtype_gps>"
  Reset Heading/1(reset) -> Logical Operator/2

== system main_RI_LIEKF_GNSSOutrage/State estimation/distribute CF/distribute CF/初始化/Subsystem ==
  sensor_data : Inport
  Enable : EnablePort
  Bus Selector1 : BusSelector  OutputSignals=IMU_Data.accl_B_m/s2_LPF,MAGN_Data.mag_norm_B
  Cross Product2 : vrlib/Utilities/Cross Product
  Cross Product3 : vrlib/Utilities/Cross Product
  Direction Cosine Matrix to Quaternions : sharedtransform/Direction Cosine Matrix  to Quaternions  aMode=aMode  action=None  tolerance=eps(2)
  Gain : Gain  Gain=-1
  Normalized1 : Subsystem
  Normalized2 : Subsystem
  Normalized3 : Subsystem
  Vector Concatenate : Concatenate  NumInputs=3  Mode=Multidimensional array  ConcatenateDimension=2
  quat_0 : Outport
  wires:
  Gain/1 -> Cross Product2/1, Cross Product3/2, Normalized3/1(fb)
  Normalized2/1(fb/g) -> Vector Concatenate/2
  Normalized3/1(fb/g) -> Vector Concatenate/3
  Cross Product2/1 -> Cross Product3/1, Normalized2/1(fb)
  Vector Concatenate/1 -> Direction Cosine Matrix to Quaternions/1
  Normalized1/1(fb/g) -> Vector Concatenate/1
  Direction Cosine Matrix to Quaternions/1 -> quat_0/1
  Bus Selector1/2 -> Cross Product2/2  "<mag_norm_B>"
  Bus Selector1/1 -> Gain/1  "<accl_B_m/s2_LPF>"
  sensor_data/1 -> Bus Selector1/1
  Cross Product3/1 -> Normalized1/1(fb)

== system main_RI_LIEKF_GNSSOutrage/Sensor_Data_Process/Magn_Data_Process1/Mag_Data_Process/Mag_Quality_Estimate/Mag_Quality/Inclination_Quality_Estimate ==
  nominal_inc_deg : Inport
  mag_normalized_O : Inport  Port=2
  Abs1 : Abs  SaturateOnIntegerOverflow=off
  Constant2 : Constant  OutDataTypeStr=Inherit: Inherit via back propagation
  Gain1 : Gain  Gain=pi/180
  Norm(x) : Subsystem
  Saturation : Saturate  UpperLimit=1  LowerLimit=0
  Selector : Selector  InputPortWidth=3  IndexOptions=Index vector (dialog)  Indices=[1 2]  OutputSizes=1
  Selector1 : Selector  InputPortWidth=3  IndexOptions=Index vector (dialog)  Indices=3  OutputSizes=1
  Subtract : Sum  Inputs=+-
  Sum3 : Sum  Inputs=+-|
  Trigonometric Function : Trigonometry  Operator=atan2
  gain : Gain  Gain=2
  inclination_quality : Outport  VectorParamsAs1DForOutWhenUnconnected=off
  wires:
  mag_normalized_O/1 -> Selector1/1, Selector/1
  Trigonometric Function/1 -> Subtract/2
  Norm(x)/1(Out1) -> Trigonometric Function/2
  Abs1/1 -> gain/1
  gain/1 -> Sum3/2
  Gain1/1 -> Subtract/1
  Subtract/1 -> Abs1/1
  Constant2/1 -> Sum3/1
  nominal_inc_deg/1 -> Gain1/1
  Sum3/1 -> Saturation/1
  Selector/1 -> Norm(x)/1(In1)
  Selector1/1 -> Trigonometric Function/1
  Saturation/1 -> inclination_quality/1

== system main_RI_LIEKF_GNSSOutrage/Sensor_Data_Process/Magn_Data_Process1/Mag_Data_Process/Mag_Quality_Estimate/Mag_Quality/Intensity_Quality_Estimate ==
  mag_normalized_O : Inport
  Abs : Abs  SaturateOnIntegerOverflow=off
  Constant1 : Constant  OutDataTypeStr=Inherit: Inherit via back propagation
  Nominal_Magnitude : Constant  OutDataTypeStr=Inherit: Inherit via back propagation
  Norm(x) : Subsystem
  Saturation : Saturate  UpperLimit=1  LowerLimit=0
  Subtract : Sum  Inputs=+-
  Sum : Sum  Inputs=+-|
  gain : Gain
  intensity_quality : Outport  VectorParamsAs1DForOutWhenUnconnected=off
  wires:
  Constant1/1 -> Sum/1
  Norm(x)/1(Out1) -> Subtract/2
  Subtract/1 -> Abs/1
  Sum/1 -> Saturation/1
  Nominal_Magnitude/1 -> Subtract/1
  Saturation/1 -> intensity_quality/1
  Abs/1 -> gain/1  "magnitude_error"
  gain/1 -> Sum/2
  mag_normalized_O/1 -> Norm(x)/1(In1)

== system main_RI_LIEKF_GNSSOutrage/Sensor_Data_Process/Magn_Data_Process1/Mag_Data_Process/Mag_Quality_Estimate/Mag_Quality/低通滤波 ==
  u : Inport
  Constant : Constant  Value=0
  Discrete-Time Integrator : DiscreteIntegrator  ExternalReset=level  SampleTime=-1  ICPrevOutput=DiscIntNeverNeededParam  ICPrevScaledInput=DiscIntNeverNeededParam
  Discrete-Time Integrator1 : DiscreteIntegrator  ExternalReset=level  InitialConditionSource=external  SampleTime=-1  ICPrevOutput=DiscIntNeverNeededParam  ICPrevScaledInput=DiscIntNeverNeededParam
  Gain : Gain  Gain=(2*pi*fc)^2
  Gain1 : Gain  Gain=2*zeta*(2*pi*fc)
  Sum : Sum  Inputs=|+-
  Sum1 : Sum  Inputs=|+-
  y : Outport
  wires:
  Sum/1 -> Gain/1
  Discrete-Time Integrator1/1 -> y/1, Sum/2
  Discrete-Time Integrator/1 -> Gain1/1, Discrete-Time Integrator1/1
  Sum1/1 -> Discrete-Time Integrator/1
  Constant/1 -> Discrete-Time Integrator1/2, Discrete-Time Integrator/2
  u/1 -> Discrete-Time Integrator1/3, Sum/1
  Gain1/1 -> Sum1/2
  Gain/1 -> Sum1/1

== system main_RI_LIEKF_GNSSOutrage/State estimation/0609bk/Error State Kalman Filter/Extended Kalman Filter1/Correct1/IGG_check ==
  Pk/k_1 : Inport
  yMeas : Inport  Port=2
  X : Inport  Port=3
  R : Inport  Port=4
  Abs : Abs  SaturateOnIntegerOverflow=off
  Abs1 : Abs  SaturateOnIntegerOverflow=off
  Add : Sum
  Add1 : Sum  Inputs=+-
  Add2 : Sum
  Constant : Constant  Value=12
  Constant1 : Constant  Value=8
  Constant2 : Constant  Value=25
  Constant3 : Constant  Value=eps
  Constant4 : Constant  Value=15
  Constant6 : Constant  Value=[eye(3),zeros(3,15)]  OutDataTypeStr=single
  Divide : Product  Inputs=*/
  Extract Diagonal1 : matrix_library/Extract Diagonal
  MATLAB Function : MATLAB Function  TreatAsAtomicUnit=on
  Product : Product  Inputs=3  Multiplication=Matrix(*)
  Product1 : Product  Multiplication=Matrix(*)
  Product2 : Product
  Scope : Scope
  Sqrt1 : Sqrt
  Transpose : Math  Operator=transpose
  yMeas1 : InportShadow  Port=2
  yMeas_out : Outport
  w : Outport  Port=2
  wires:
  Product/1 -> Add/1
  Transpose/1 -> Product/3
  R/1 -> Add/2
  Pk/k_1/1 -> Product/2
  yMeas/1 -> Add1/1
  Constant6/1 -> Product1/1, Product/1, Transpose/1
  X/1 -> Product1/2
  Product1/1 -> Add1/2
  Product2/1 -> yMeas_out/1
  Add/1 -> Extract Diagonal1/1  "S"
  Divide/1 -> Abs/1, Scope/1
  MATLAB Function/1(w) -> w/1, Product2/1
  Extract Diagonal1/1 -> Abs1/1
  Add1/1 -> Divide/1
  Sqrt1/1 -> Add2/1
  Abs/1 -> MATLAB Function/1(err)
  Abs1/1 -> Sqrt1/1
  Add2/1 -> Divide/2
  Constant3/1 -> Add2/2
  yMeas1/1 -> Product2/2
  Constant1/1 -> MATLAB Function/2(k0)
  Constant4/1 -> MATLAB Function/3(k1)
  Constant/1 -> MATLAB Function/4(zk0)
  Constant2/1 -> MATLAB Function/5(zk1)

== system main_RI_LIEKF_GNSSOutrage/State estimation/0609bk/Error State Kalman Filter/Extended Kalman Filter1/Predict/If Action Subsystem ==
  Action Port : ActionPort
  Constant : Constant  Value=0
  Data Store Read : DataStoreRead  DataStoreName=x  IndexOptions=Index vector (dialog)  Indices=1  OutputSizes=1
  Data Store Write : DataStoreWrite  DataStoreName=x  IndexOptions=Index vector (dialog)  Indices=1  OutputSizes=1
  Data Store Write1 : DataStoreWrite  DataStoreName=feedback_flag_18dim  IndexOptions=Index vector (dialog)  Indices=1  OutputSizes=1
  Mux : Mux  Inputs=2
  Selector : Selector  InputPortWidth=18  IndexOptions=Index vector (dialog)  Indices=[16 17 18]  OutputSizes=1
  Zero : Constant  Value=zeros(15,1)  OutDataTypeStr=Inherit: Inherit via back propagation
  wires:
  Mux/1 -> Data Store Write/1
  Selector/1 -> Mux/2
  Zero/1 -> Mux/1
  Data Store Read/1 -> Selector/1
  Constant/1 -> Data Store Write1/1

== system main_RI_LIEKF_GNSSOutrage/State estimation/0609bk/INS propogation/Init_PVQ/Horizontal_attitude/Deal with zero ==
  In1 : Inport
  Add5 : Sum
  Constant1 : Constant  Value=1e-6  OutDataTypeStr=single
  Out1 : Outport
  wires:
  Add5/1 -> Out1/1
  In1/1 -> Add5/1
  Constant1/1 -> Add5/2

== system main_RI_LIEKF_GNSSOutrage/State estimation/15dim KF1/Error State Kalman Filter/GNSS//INS Kalman Filter1/CovarianceOutputConfigurator/decideOutput ==
  Z : Inport
  SqrtUsedFcn : MATLAB Function  TreatAsAtomicUnit=on
  isSqrtUsed : Constant  Value=pInitialization.isSqrtUsed  VectorParams1D=off  OutDataTypeStr=boolean
  P : Outport
  wires:
  SqrtUsedFcn/1(P) -> P/1
  Z/1 -> SqrtUsedFcn/1(u)
  isSqrtUsed/1 -> SqrtUsedFcn/2(isSqrtUsed)

== system main_RI_LIEKF_GNSSOutrage/State estimation/15dim KF1/Error State Kalman Filter/GNSS//INS Kalman Filter1/Observer/MeasurementUpdate ==
  L[k] : Inport
  y[k] : Inport  Port=2
  C[k] : Inport  Port=3
  xhat[k|k-1] : Inport  Port=4
  D[k] : Inport  Port=5
  u[k] : Inport  Port=6
  Enable : EnablePort
  Add1 : Sum
  C[k]*xhat[k|k-1] : Product  Multiplication=Matrix(*)
  D[k]*u[k] : Product  Multiplication=Matrix(*)
  Product3 : Product  Multiplication=Matrix(*)
  Sum : Sum  Inputs=|+-
  L*(y[k]-yhat[k|k-1]) : Outport  OutputWhenDisabled=reset  InitialOutput=0  VectorParamsAs1DForOutWhenUnconnected=off
  wires:
  u[k]/1 -> D[k]*u[k]/2
  D[k]/1 -> D[k]*u[k]/1
  xhat[k|k-1]/1 -> C[k]*xhat[k|k-1]/2
  C[k]/1 -> C[k]*xhat[k|k-1]/1
  C[k]*xhat[k|k-1]/1 -> Add1/1
  D[k]*u[k]/1 -> Add1/2
  Add1/1 -> Sum/2  "yhat[k|k-1]"
  Sum/1 -> Product3/2
  y[k]/1 -> Sum/1
  Product3/1 -> L*(y[k]-yhat[k|k-1])/1
  L[k]/1 -> Product3/1

== system main_RI_LIEKF_GNSSOutrage/State estimation/15dim KF1/INS propogation/Init_PVQ2/Horizontal_attitude/Deal with zero ==
  In1 : Inport
  Add5 : Sum
  Constant1 : Constant  Value=1e-6  OutDataTypeStr=single
  Out1 : Outport
  wires:
  Constant1/1 -> Add5/2
  In1/1 -> Add5/1
  Add5/1 -> Out1/1

== system main_RI_LIEKF_GNSSOutrage/State estimation/15dim KF1/INS propogation/gyro bias compensation/error compensation/If Action Subsystem1 ==
  Action Port : ActionPort
  Constant : Constant
  Data Store Write : DataStoreWrite  DataStoreName=feedback_flag  IndexOptions=Index vector (dialog)  Indices=1  OutputSizes=1
  wires:
  Constant/1 -> Data Store Write/1

== system main_RI_LIEKF_GNSSOutrage/State estimation/ER EKF/Error State Kalman Filter/Extended Kalman Filter1/Predict/If Action Subsystem ==
  Action Port : ActionPort
  Constant : Constant  Value=0
  Data Store Read : DataStoreRead  DataStoreName=x  IndexOptions=Index vector (dialog)  Indices=1  OutputSizes=1
  Data Store Write : DataStoreWrite  DataStoreName=x  IndexOptions=Index vector (dialog)  Indices=1  OutputSizes=1
  Data Store Write1 : DataStoreWrite  DataStoreName=feedback_flag_18dim  IndexOptions=Index vector (dialog)  Indices=1  OutputSizes=1
  Mux : Mux  Inputs=2
  Selector : Selector  InputPortWidth=18  IndexOptions=Index vector (dialog)  Indices=[16 17 18]  OutputSizes=1
  Zero : Constant  Value=zeros(15,1)  OutDataTypeStr=Inherit: Inherit via back propagation
  wires:
  Constant/1 -> Data Store Write1/1
  Data Store Read/1 -> Selector/1
  Zero/1 -> Mux/1
  Selector/1 -> Mux/2
  Mux/1 -> Data Store Write/1

== system main_RI_LIEKF_GNSSOutrage/State estimation/ER EKF/INS propogation/Init_PVQ/Horizontal_attitude/Deal with zero ==
  In1 : Inport
  Add5 : Sum
  Constant1 : Constant  Value=1e-6  OutDataTypeStr=single
  Out1 : Outport
  wires:
  Constant1/1 -> Add5/2
  In1/1 -> Add5/1
  Add5/1 -> Out1/1

== system main_RI_LIEKF_GNSSOutrage/State estimation/ER EKF/INS propogation/Init_PVQ/Horizontal_attitude2/Deal with zero ==
  In1 : Inport
  Add5 : Sum
  Constant1 : Constant  Value=1e-6  OutDataTypeStr=single
  Out1 : Outport
  wires:
  Constant1/1 -> Add5/2
  In1/1 -> Add5/1
  Add5/1 -> Out1/1

== system main_RI_LIEKF_GNSSOutrage/State estimation/ER EKF/INS propogation/gyro bias compensation/error compensation/If Action Subsystem1 ==
  Action Port : ActionPort  ActionPortLabel=if(u1 == 1)
  Constant : Constant
  Data Store Write : DataStoreWrite  DataStoreName=feedback_flag_18dim  IndexOptions=Index vector (dialog)  Indices=1  OutputSizes=1
  wires:
  Constant/1 -> Data Store Write/1

== system main_RI_LIEKF_GNSSOutrage/State estimation/LI EKF2/Error State Kalman Filter/Extended Kalman Filter1/Correct1/IGG_check ==
  Pk/k_1 : Inport
  yMeas : Inport  Port=2
  X : Inport  Port=3
  R : Inport  Port=4
  Abs : Abs  Commented=on  SaturateOnIntegerOverflow=off
  Abs1 : Abs  Commented=on  SaturateOnIntegerOverflow=off
  Add : Sum  Commented=on
  Add1 : Sum  Inputs=+-
  Add2 : Sum  Commented=on
  Constant : Constant  Commented=on  Value=12
  Constant1 : Constant  Commented=on  Value=8
  Constant2 : Constant  Value=25
  Constant3 : Constant  Commented=on  Value=eps
  Constant4 : Constant  Commented=on  Value=15
  Constant6 : Constant  Value=[zeros(6,3),eye(6),zeros(6,6)]  OutDataTypeStr=single
  Divide : Product  Commented=on  Inputs=*/
  Extract Diagonal1 : matrix_library/Extract Diagonal  Commented=on
  MATLAB Function : MATLAB Function  Commented=on  TreatAsAtomicUnit=on
  Product : Product  Inputs=3  Multiplication=Matrix(*)
  Product1 : Product  Multiplication=Matrix(*)
  Product2 : Product
  Scope : Scope  Commented=on
  Sqrt1 : Sqrt  Commented=on
  Transpose : Math  Operator=transpose
  yMeas1 : InportShadow  Port=2
  yMeas_out : Outport
  w : Outport  Port=2
  inno : Outport  Port=3
  wires:
  Product/1 -> Add/1
  Transpose/1 -> Product/3
  R/1 -> Add/2
  Pk/k_1/1 -> Product/2
  yMeas/1 -> Add1/1
  Constant6/1 -> Product1/1, Product/1, Transpose/1
  X/1 -> Product1/2
  Product1/1 -> Add1/2
  Product2/1 -> yMeas_out/1
  Add/1 -> Extract Diagonal1/1  "S"
  Divide/1 -> Abs/1, Scope/1
  MATLAB Function/1(w) -> w/1, Product2/1
  Extract Diagonal1/1 -> Abs1/1
  Add1/1 -> inno/1, Divide/1
  Sqrt1/1 -> Add2/1
  Abs/1 -> MATLAB Function/1(err)
  Abs1/1 -> Sqrt1/1
  Add2/1 -> Divide/2
  Constant3/1 -> Add2/2
  yMeas1/1 -> Product2/2
  Constant1/1 -> MATLAB Function/2(k0)
  Constant4/1 -> MATLAB Function/3(k1)
  Constant/1 -> MATLAB Function/4(zk0)
  Constant2/1 -> MATLAB Function/5(zk1)

== system main_RI_LIEKF_GNSSOutrage/State estimation/LI EKF2/Error State Kalman Filter/Extended Kalman Filter1/Predict/If Action Subsystem ==
  Action Port : ActionPort
  Constant : Constant  Value=0
  Data Store Read : DataStoreRead  DataStoreName=x  IndexOptions=Index vector (dialog)  Indices=1  OutputSizes=1
  Data Store Write : DataStoreWrite  DataStoreName=x  IndexOptions=Index vector (dialog)  Indices=1  OutputSizes=1
  Data Store Write1 : DataStoreWrite  DataStoreName=feedback_flag_18dim  IndexOptions=Index vector (dialog)  Indices=1  OutputSizes=1
  Mux : Mux  Inputs=2
  Selector : Selector  InputPortWidth=18  IndexOptions=Index vector (dialog)  Indices=[16 17 18]  OutputSizes=1
  Zero : Constant  Value=zeros(15,1)  OutDataTypeStr=Inherit: Inherit via back propagation
  wires:
  Mux/1 -> Data Store Write/1
  Selector/1 -> Mux/2
  Zero/1 -> Mux/1
  Data Store Read/1 -> Selector/1
  Constant/1 -> Data Store Write1/1

== system main_RI_LIEKF_GNSSOutrage/State estimation/LI EKF2/Error State Kalman Filter/bak/Simulink Function - State Transition Jacobian/Cal Phi1 ==
  Rbn : Inport
  vn : Inport  Port=2
  pn : Inport  Port=3
  Constant : Constant  Value=dt
  MATLAB Function1 : MATLAB Function  TreatAsAtomicUnit=on
  Reshape : Reshape  OutputDimensionality=Column vector (2-D)
  Reshape1 : Reshape  OutputDimensionality=Column vector (2-D)
  Phi : Outport
  wires:
  Constant/1 -> MATLAB Function1/4(dt)
  MATLAB Function1/1(Phi) -> Phi/1
  Rbn/1 -> MATLAB Function1/3(Rbn)
  vn/1 -> Reshape/1
  pn/1 -> Reshape1/1
  Reshape/1 -> MATLAB Function1/1(vn)
  Reshape1/1 -> MATLAB Function1/2(pn)

== system main_RI_LIEKF_GNSSOutrage/State estimation/LI EKF2/INS propogation/AOA//SA//Vwind update/Subsystem/LSTM predict ==
  X : Inport
  Data Type Conversion11 : DataTypeConversion  OutDataTypeStr=double  SaturateOnIntegerOverflow=off  RndMeth=Floor
  MATLAB Function5 : MATLAB Function  TreatAsAtomicUnit=on
  MATLAB Function6 : MATLAB Function  TreatAsAtomicUnit=on
  Predict : deeplib/Predict  Network=Network from MAT-file  NetworkFunction=squeezenet  NetworkFilePath=D:\app\RIEKFModel\lstmnet.mat  MiniBatchSize=128  InputDataFormats={'',''}  Predictions=on  Activations={}  ForceInterpretedSim=off  EnableDLNetwork=on
  Transpose2 : Math  Operator=transpose
  YPred_test_out : Outport
  wires:
  Predict/1 -> MATLAB Function6/1(YPred_test)
  Transpose2/1 -> Predict/1
  MATLAB Function6/1(YPred_test_out) -> YPred_test_out/1
  Data Type Conversion11/1 -> MATLAB Function5/1(X)
  X/1 -> Data Type Conversion11/1
  MATLAB Function5/1(X_nYPred) -> Transpose2/1

== system main_RI_LIEKF_GNSSOutrage/State estimation/LI EKF2/INS propogation/AOA//SA//Vwind update/Subsystem/LSTM predict1 ==
  X : Inport
  Data Type Conversion11 : DataTypeConversion  OutDataTypeStr=double  SaturateOnIntegerOverflow=off  RndMeth=Floor
  MATLAB Function5 : MATLAB Function  TreatAsAtomicUnit=on
  MATLAB Function6 : MATLAB Function  TreatAsAtomicUnit=on
  Predict : deeplib/Predict  Network=Network from MAT-file  NetworkFunction=squeezenet  NetworkFilePath=D:\app\RIEKFModel\lstmnetSA.mat  MiniBatchSize=128  InputDataFormats={'',''}  Predictions=on  Activations={}  ForceInterpretedSim=off  EnableDLNetwork=on
  Transpose2 : Math  Operator=transpose
  YPred_test_out : Outport
  wires:
  MATLAB Function5/1(X_nYPred) -> Transpose2/1
  X/1 -> Data Type Conversion11/1
  Data Type Conversion11/1 -> MATLAB Function5/1(X)
  MATLAB Function6/1(YPred_test_out) -> YPred_test_out/1
  Transpose2/1 -> Predict/1
  Predict/1 -> MATLAB Function6/1(YPred_test)

== system main_RI_LIEKF_GNSSOutrage/State estimation/LI EKF2/INS propogation/AOA//SA//Vwind update/Subsystem/Subsystem ==
  In1 : Inport
  v : Inport  Port=2
  Asin : Trigonometry  Operator=asin
  Math Function : Math  Operator=magnitude^2
  Product1 : Product
  Reciprocal Sqrt : Sqrt  Operator=rSqrt
  Sum of Elements : Sum  Inputs=+
  beta : Outport
  wires:
  Product1/1 -> Asin/1
  Sum of Elements/1 -> Reciprocal Sqrt/1
  Math Function/1 -> Sum of Elements/1
  Reciprocal Sqrt/1 -> Product1/1
  Asin/1 -> beta/1  "beta"
  In1/1 -> Math Function/1
  v/1 -> Product1/2

== system main_RI_LIEKF_GNSSOutrage/State estimation/LI EKF2/INS propogation/Init_PVQ/Horizontal_attitude1/Deal with zero ==
  In1 : Inport
  Add5 : Sum
  Constant1 : Constant  Value=1e-6  OutDataTypeStr=single
  Out1 : Outport
  wires:
  Constant1/1 -> Add5/2
  In1/1 -> Add5/1
  Add5/1 -> Out1/1

== system main_RI_LIEKF_GNSSOutrage/State estimation/LI EKF2/INS propogation/Init_PVQ/Horizontal_attitude2/Deal with zero ==
  In1 : Inport
  Add5 : Sum
  Constant1 : Constant  Value=1e-6  OutDataTypeStr=single
  Out1 : Outport
  wires:
  Constant1/1 -> Add5/2
  In1/1 -> Add5/1
  Add5/1 -> Out1/1

== system main_RI_LIEKF_GNSSOutrage/State estimation/LI EKF2/INS propogation/gyro bias compensation/error compensation/If Action Subsystem1 ==
  Action Port : ActionPort
  Constant : Constant
  Data Store Write : DataStoreWrite  DataStoreName=feedback_flag_18dim_LIEKF  IndexOptions=Index vector (dialog)  Indices=1  OutputSizes=1
  wires:
  Constant/1 -> Data Store Write/1

== system main_RI_LIEKF_GNSSOutrage/State estimation/RI EKF_AOA_LSTM/Error State Kalman Filter/Extended Kalman Filter1/Correct1/IGG_check ==
  Pk/k_1 : Inport
  yMeas : Inport  Port=2
  X : Inport  Port=3
  R : Inport  Port=4
  Abs : Abs  Commented=on  SaturateOnIntegerOverflow=off
  Abs1 : Abs  Commented=on  SaturateOnIntegerOverflow=off
  Add : Sum  Commented=on
  Add1 : Sum  Inputs=+-
  Add2 : Sum  Commented=on
  Constant : Constant  Commented=on  Value=12
  Constant1 : Constant  Commented=on  Value=8
  Constant2 : Constant  Value=25
  Constant3 : Constant  Commented=on  Value=eps
  Constant4 : Constant  Commented=on  Value=15
  Constant6 : Constant  Value=[zeros(6,3),eye(6),zeros(6,6)]  OutDataTypeStr=single
  Divide : Product  Commented=on  Inputs=*/
  Extract Diagonal1 : matrix_library/Extract Diagonal  Commented=on
  MATLAB Function : MATLAB Function  Commented=on  TreatAsAtomicUnit=on
  Product : Product  Inputs=3  Multiplication=Matrix(*)
  Product1 : Product  Multiplication=Matrix(*)
  Product2 : Product
  Scope : Scope  Commented=on
  Sqrt1 : Sqrt  Commented=on
  Transpose : Math  Operator=transpose
  yMeas1 : InportShadow  Port=2
  yMeas_out : Outport
  w : Outport  Port=2
  inno : Outport  Port=3
  wires:
  Product/1 -> Add/1
  Transpose/1 -> Product/3
  R/1 -> Add/2
  Pk/k_1/1 -> Product/2
  yMeas/1 -> Add1/1
  Constant6/1 -> Product1/1, Product/1, Transpose/1
  X/1 -> Product1/2
  Product1/1 -> Add1/2
  Product2/1 -> yMeas_out/1
  Add/1 -> Extract Diagonal1/1  "S"
  Divide/1 -> Abs/1, Scope/1
  MATLAB Function/1(w) -> w/1, Product2/1
  Extract Diagonal1/1 -> Abs1/1
  Add1/1 -> inno/1, Divide/1
  Sqrt1/1 -> Add2/1
  Abs/1 -> MATLAB Function/1(err)
  Abs1/1 -> Sqrt1/1
  Add2/1 -> Divide/2
  Constant3/1 -> Add2/2
  yMeas1/1 -> Product2/2
  Constant1/1 -> MATLAB Function/2(k0)
  Constant4/1 -> MATLAB Function/3(k1)
  Constant/1 -> MATLAB Function/4(zk0)
  Constant2/1 -> MATLAB Function/5(zk1)

== system main_RI_LIEKF_GNSSOutrage/State estimation/RI EKF_AOA_LSTM/Error State Kalman Filter/Extended Kalman Filter1/Predict/If Action Subsystem ==
  Action Port : ActionPort
  Constant : Constant  Value=0
  Data Store Read : DataStoreRead  DataStoreName=x  IndexOptions=Index vector (dialog)  Indices=1  OutputSizes=1
  Data Store Write : DataStoreWrite  DataStoreName=x  IndexOptions=Index vector (dialog)  Indices=1  OutputSizes=1
  Data Store Write1 : DataStoreWrite  DataStoreName=feedback_flag_18dim  IndexOptions=Index vector (dialog)  Indices=1  OutputSizes=1
  Mux : Mux  Inputs=2
  Selector : Selector  InputPortWidth=18  IndexOptions=Index vector (dialog)  Indices=[16 17 18]  OutputSizes=1
  Zero : Constant  Value=zeros(15,1)  OutDataTypeStr=Inherit: Inherit via back propagation
  wires:
  Mux/1 -> Data Store Write/1
  Selector/1 -> Mux/2
  Zero/1 -> Mux/1
  Data Store Read/1 -> Selector/1
  Constant/1 -> Data Store Write1/1
